simulink model "altitude_hold_using_commanded_pitch"  (Simulink 7.7)
settings: Solver=ode45  StartTime=0.0  StopTime=10.0  RelTol=1e-3
undefined symbols (not defined in the file): k_i_h, k_p_h, Va
settings Model: Creator=prattmic  LastModifiedBy=prattmic

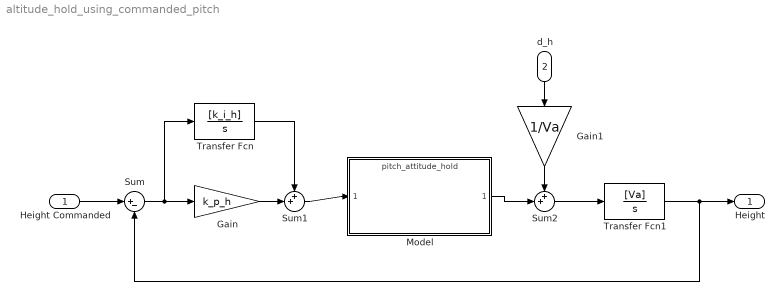
== system altitude_hold_using_commanded_pitch ==
  Height Commanded : Inport
  d_h : Inport  Port=2
  Gain : Gain  Gain=k_p_h
  Gain1 : Gain  Gain=1/Va
  Model : ModelReference  ModelNameDialog=pitch_attitude_hold  SimulationMode=Normal  ModelReferenceVersion=1.6  CopyOfModelName=pitch_attitude_hold  DefaultDataLogging=on
  Sum : Sum  Inputs=|+-
  Sum1 : Sum  Inputs=++|
  Sum2 : Sum  Inputs=++|
  Transfer Fcn : TransferFcn  Numerator=[k_i_h]  Denominator=[1 0]
  Transfer Fcn1 : TransferFcn  Numerator=[Va]  Denominator=[1 0]
  Height : Outport
  wires:
  Height Commanded/1 -> Sum/1
  Sum/1 -> Gain/1, Transfer Fcn/1
  Sum1/1 -> Model/1
  Transfer Fcn/1 -> Sum1/1
  Gain/1 -> Sum1/2
  Transfer Fcn1/1 -> Height/1, Sum/2
  d_h/1 -> Gain1/1
  Gain1/1 -> Sum2/1
  Sum2/1 -> Transfer Fcn1/1
  Model/1 -> Sum2/2
